simulink model "CAMFC2_Quad_New_02_Payload_01"  (R2018b)
settings: Solver=ode45  StartTime=0.0  StopTime=200  RelTol=1e-3  EnableMultiTasking=on
InitFcn:
  | constant_CAMFC2_Quad_New_02_Payload_01
values from neighbouring files (symbols this model uses):
  alpha = 0.01    [constant_CAMFC2_Quad_New_02_Payload_01.m]
  AN = [     0 1 0 0 ... (first row only)    [constant_CAMFC2_Quad_New_02_Payload_01.m]
  B = 1e0*eye(n)    [Simple_2Quad_payload_03_const.m]    (also in constant_CAMFC2_Quad_New_02_Payload_01.m = eye(n); test01.m = [eye(3) eye(3) eye(3) eye(3))
  B_pseudo_inverse = ((B'*B)^(-1))*B'    [constant_CAMFC2_Quad_New_02_Payload_01.m]
  BBT_inv = ((B'*B)^(-1))*B'    [Simple_2Quad_payload_03_const.m]    (also in Simple_4Quad_payload_04_const.m = ((BR'*BR)^(-1))*BR'; Simple_4Quad_payload_05_const.m = ((BR'*BR)^(-1))*BR'; Simple_4Quad_payload_06_const.m = ((BR'*BR)^(-1))*BR'; Simple_4Quad_payload_07_const.m = ((BR'*BR)^(-1))*BR')
  Beta = 0.1    [constant_CAMFC2_Quad_New_02_Payload_01.m]
  BN = [     1 0 0 0 ... (first row only)    [constant_CAMFC2_Quad_New_02_Payload_01.m]
  epsilon_struct = struct('data',epsilon_InitVal)    [constant_CAMFC2_Quad_New_02_Payload_01.m]
  gama1 = 1e+3*diag([1e-6*ones(n0,1);1e-0*ones(n0,1)])    [constant_CAMFC2_Quad_New_02_Payload_01.m]
  gama2 = 1e-1*diag([1e-6*ones(n0,1);1e-0*ones(n0,1)])    [constant_CAMFC2_Quad_New_02_Payload_01.m]
  gamma_0 = 1e-0*diag([1e-3;1e-0])    [Simple_2Quad_payload_03_const.m]    (also in Simple_4Quad_payload_04_const.m = 1e-0*diag([1e-6*ones(3,1);1e-0*ones(3,1)]); Simple_4Quad_payload_05_const.m = 1e-1*diag([1e-6*ones(3,1);1e-0*ones(3,1)]); Simple_4Quad_payload_06_const.m = 1e-0*diag([1e-6*ones(3,1);1e-0*ones(3,1)]); Simple_4Quad_payload_07_const.m = 1e-0*diag([1e-6*ones(3,1);1e-0*ones(3,1)]))
  gamma_1 = 1e+2*diag([1e-3;1e-0])    [Simple_2Quad_payload_03_const.m]    (also in Simple_4Quad_payload_04_const.m = 1e+2*diag([1e-6*ones(3,1);1e-0*ones(3,1)]); Simple_4Quad_payload_05_const.m = 1e+2*diag([1e-6*ones(3,1);1e-0*ones(3,1)]); Simple_4Quad_payload_06_const.m = 1e+3*diag([1e-6*ones(3,1);1e-0*ones(3,1)]); Simple_4Quad_payload_07_const.m = 1e+3*diag([1e-6*ones(3,1);1e-0*ones(3,1)]))
  ge = 9.81    [Simple_4Quad_payload_03_const.m]    (also in constant_CAMFC2_Quad_New_02_Payload_01.m)
  H = L + BN    [constant_CAMFC2_Quad_New_02_Payload_01.m]
  J = 1.2416e-3 * diag([1 1 2],0)    [constant_CAMFC2_Quad_New_02_Payload_01.m]
  K = 1e+1*eye(n)    [constant_CAMFC2_Quad_New_02_Payload_01.m]
  k1 = 1    [Simple_2Quad_payload_03_const.m]    (also in Simple_4Quad_payload_04_const.m; Simple_4Quad_payload_05_const.m; Simple_4Quad_payload_06_const.m; Simple_4Quad_payload_07_const.m)
  k2 = 0.1    [Simple_2Quad_payload_03_const.m]    (also in Simple_4Quad_payload_04_const.m; Simple_4Quad_payload_05_const.m; Simple_4Quad_payload_06_const.m; Simple_4Quad_payload_07_const.m)
  Ka = 0.01    [Simple_4Quad_payload_03_const.m]    (also in constant_CAMFC2_Quad_New_02_Payload_01.m)
  Kd = 0.01    [Simple_4Quad_payload_03_const.m]    (also in constant_CAMFC2_Quad_New_02_Payload_01.m)
  Kf = 1.0e-5    (= 1e-05)    [Simple_4Quad_payload_03_const.m]    (also in constant_CAMFC2_Quad_New_02_Payload_01.m)
  Kt = 0.0435 * Kf    (= 4.35e-07)    [Simple_4Quad_payload_03_const.m]    (also in constant_CAMFC2_Quad_New_02_Payload_01.m = 1e-07)
  Lq = 0.45    [Simple_4Quad_payload_03_const.m]    (also in constant_CAMFC2_Quad_New_02_Payload_01.m = 0.2)
  m = 1.5    [Colab_4Quad_model_01_const.m]    (also in Colab_4Quad_model_02_const.m; Simple_2Quad_payload_04_const.m = 1; Simple_4Quad_payload_01_const.m = 1; Simple_4Quad_payload_02_const.m = 1)
  M = 1.0    (= 1)    [Colab_4Quad_model_01_const.m]    (also in Colab_4Quad_model_02_const.m; Simple_2Quad_payload_01_const.m; Simple_2Quad_payload_02_const.m; Simple_2Quad_payload_03_const.m)
  mp = 10    [constant_CAMFC2_Quad_New_02_Payload_01.m]
  N = 4    [constant_CAMFC2_Quad_New_02_Payload_01.m]
  n = 2    [Simple_2Quad_payload_03_const.m]    (also in Simple_4Quad_payload_03_const.m = 6; Simple_4Quad_payload_04_const.m = 6; Simple_4Quad_payload_05_const.m = 6; Simple_4Quad_payload_06_const.m = 6)
  n0 = 3    [constant_CAMFC2_Quad_New_02_Payload_01.m]
  np = 3    [Simple_4Quad_payload_10_const.m]    (also in Simple_4Quad_payload_11_const.m; Simple_4Quad_payload_12_const.m; constant_CAMFC2_Quad_New_02_Payload_01.m = 6)
  Observer_Gain = 10    [constant_CAMFC2_Quad_New_02_Payload_01.m]
  Observer_Gain1 = 10    [constant_CAMFC2_Quad_New_02_Payload_01.m]
  P_struct = struct('data',P_InitVal)    [constant_CAMFC2_Quad_New_02_Payload_01.m]
  Q = 1e-1*eye(n)    [Simple_2Quad_payload_03_const.m]    (also in constant_CAMFC2_Quad_New_02_Payload_01.m = 1e+1*eye(n))
  QR = 1e-0*eye(n)    [Simple_4Quad_payload_04_const.m]    (also in Simple_4Quad_payload_05_const.m = 1e-1*eye(n); Simple_4Quad_payload_06_const.m; Simple_4Quad_payload_07_const.m; Simple_4Quad_payload_08_const.m)
  R = 1e+0*eye(n)    [Simple_2Quad_payload_03_const.m]    (also in Simple_4Quad_payload_04_const.m = 1e+0*eye(m); Simple_4Quad_payload_05_const.m = 1e+0*eye(m); Simple_4Quad_payload_06_const.m; Simple_4Quad_payload_07_const.m)
  r_formX = 1.0    (= 1)    [constant_CAMFC2_Quad_New_02_Payload_01.m]
  r_formY = 1.0    (= 1)    [constant_CAMFC2_Quad_New_02_Payload_01.m]
  r_formZ = 1.0    (= 1)    [constant_CAMFC2_Quad_New_02_Payload_01.m]
  rho1 = 1e-0    (= 1)    [constant_CAMFC2_Quad_New_02_Payload_01.m]
  rho2 = 1e-1    (= 0.1)    [constant_CAMFC2_Quad_New_02_Payload_01.m]
  rho_0 = 1e-0    (= 1)    [Simple_2Quad_payload_03_const.m]    (also in Simple_4Quad_payload_04_const.m; Simple_4Quad_payload_05_const.m = 0.1; Simple_4Quad_payload_06_const.m; Simple_4Quad_payload_07_const.m)
  rho_1 = 1e-0    (= 1)    [Simple_2Quad_payload_03_const.m]    (also in Simple_4Quad_payload_04_const.m; Simple_4Quad_payload_05_const.m; Simple_4Quad_payload_06_const.m; Simple_4Quad_payload_07_const.m)
  T_struct = struct('data',T_InitVal)    [constant_CAMFC2_Quad_New_02_Payload_01.m]
  U_dot0_M = U_dot0_m*ones(n0,1)    [constant_CAMFC2_Quad_New_02_Payload_01.m]
  Upsilon_M = Upsilon_m*ones(n0,1)    [constant_CAMFC2_Quad_New_02_Payload_01.m]
  X_M = X_m*ones(n0,1)    [constant_CAMFC2_Quad_New_02_Payload_01.m]
(part 1 of 3)
settings Model: ExtModeTrigDuration=100  Creator=hp  LastModifiedBy=ali
settings DataIOCC: LimitDataPoints=on  SaveFinalState=on  SaveFormat=StructureWithTime  SaveOutput=off  SaveState=on  StateSaveName=tmp_raccel_xout  SignalLoggingName=tmp_raccel_logsout
settings OptimizationCC: EfficientMapNaN2IntZero=off  LifeSpan=inf
settings DebuggingCC: UnderspecifiedInitializationDetection=Classic  MergeDetectMultiDrivingBlocksExec=none  SFUnexpectedBacktrackingDiag=warning  SFNoUnconditionalDefaultTransitionDiag=warning  SFExecutionAtInitializationDiag=none
settings HardwareCC: ProdBitPerPointer=32  ProdBitPerSizeT=32  ProdBitPerPtrDiffT=32  ProdLargestAtomicFloat=None  ProdIntDivRoundTo=Undefined  ProdEndianess=Unspecified  ProdWordSize=32  ProdHWDeviceType=32-bit Generic  TargetBitPerPointer=64  TargetBitPerSizeT=64  TargetBitPerPtrDiffT=64  TargetLongLongMode=on  TargetIntDivRoundTo=Zero  TargetEndianess=LittleEndian  TargetWordSize=64  TargetHWDeviceType=MATLAB Host  ProdEqTarget=off
settings ModelReferenceCC: PropagateSignalLabelsOutOfModel=off
settings SFSimCC: SimUseLocalCustomCode=off
settings RTWCC: SystemTargetFile=raccel.tlc  TemplateMakefile=raccel_default_tmf  RTWVerbose=off  RTWUseLocalCustomCode=off  RTWUseSimCustomCode=on
settings CodeAppCC: GenerateComments=off  MaxIdLength=128  MangleLength=10  SimulinkBlockComments=off
settings RaccelTargetCC: GeneratePreprocessorConditionals=Use local settings  MultiInstanceERTCode=off  PreserveStateflowLocalDataDimensions=off  ExtModeMexArgs='', 0, 54523  ENABLE_SLEXEC_SSBRIDGE=0  RTWCAPIParams=on
settings ConfigComp: CovMetricSettings=dw  CovHtmlReporting=on  CovSaveCumulativeToWorkspaceVar=on  CovSaveSingleToWorkspaceVar=on  CovExternalEMLEnable=off

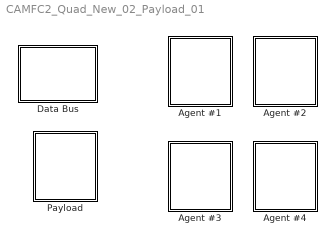
== system CAMFC2_Quad_New_02_Payload_01 ==
  Agent #1 : Subsystem
  Agent #2 : Subsystem
  Agent #3 : Subsystem
  Agent #4 : Subsystem
  "Data Bus " : Subsystem
  Payload : Subsystem

== system CAMFC2_Quad_New_02_Payload_01/Agent #1 ==
  Agent # : Constant
  Controller #1 : Subsystem
  Plant #1 : Subsystem
  tag scope: x1=global
  wires:
  Plant #1/1(X) -> [x1]
  Controller #1/1(u1) -> Plant #1/1(U)
  Agent #/1 -> Controller #1/1(Agent No.)

== system CAMFC2_Quad_New_02_Payload_01/Agent #2 ==
  Agent # : Constant  Value=2
  Controller #2 : Subsystem
  Plant #2 : Subsystem
  tag scope: x2=global
  wires:
  Plant #2/1(X) -> [x2]
  Controller #2/1(u2) -> Plant #2/1(U)
  Agent #/1 -> Controller #2/1(Agent No.)

== system CAMFC2_Quad_New_02_Payload_01/Agent #3 ==
  Agent # : Constant  Value=3
  Controller #3 : Subsystem
  Plant #3 : Subsystem
  tag scope: x3=global
  wires:
  Plant #3/1(X) -> [x3]
  Controller #3/1(u3) -> Plant #3/1(U)
  Agent #/1 -> Controller #3/1(Agent No.)

== system CAMFC2_Quad_New_02_Payload_01/Agent #4 ==
  Agent # : Constant  Value=4
  Controller #4 : Subsystem
  Plant #4 : Subsystem
  tag scope: x4=global
  wires:
  Plant #4/1(X) -> [x4]
  Controller #4/1(u4) -> Plant #4/1(U)
  Agent #/1 -> Controller #4/1(Agent No.)

== system CAMFC2_Quad_New_02_Payload_01/Data Bus  ==
  Mux6 : Mux
  Observers Log : Subsystem
  Reference Trajectory : Subsystem
  Rotational Log : Subsystem
  Scope{1..2,16..19,25..26} (8 alike) : Scope
  Sum : Sum  Inputs=|-+
  Translational Log : Subsystem
  formation of the leader : Constant  Value=zeros(n0,1)
  tag scope: u0=global, x0=global, x=global, z0=global
  wires:
  Reference Trajectory/2(U0) -> [u0], Scope25/1
  Reference Trajectory/1(X0) -> [x0], Sum/1, Scope26/1
  [x2] -> Scope17/1, Mux6/2
  [x1] -> Scope16/1, Mux6/1
  Mux6/1 -> [x]
  [x3] -> Scope18/1, Mux6/3
  [x4] -> Mux6/4, Scope19/1
  formation of the leader/1 -> Sum/2
  Sum/1 -> [z0]
  [x_p] -> Scope1/1
  [u_p] -> Scope2/1

== system CAMFC2_Quad_New_02_Payload_01/Payload ==
  "Controller " : Subsystem
  Plant : Subsystem
  tag scope: u_p=global, x_p=global
  wires:
  "Controller "/1(u) -> [u_p], Plant/1(U)
  Plant/1(X) -> "Controller "/1(X), [x_p]

== system CAMFC2_Quad_New_02_Payload_01/Agent #1/Controller #1 ==
  Agent No. : Inport
  Controller Interpreter #1 : MATLAB Function  TreatAsAtomicUnit=on
  Controller to Motors #1 : MATLAB Function  TreatAsAtomicUnit=on
  Cooperative Observers #1 : Subsystem
  Demux : Demux  Outputs=2
  Rotational : Subsystem
  Scope : Scope
  Sum : Sum  Inputs=|++
  Translational #1 : Subsystem
  u1 : Outport
  tag scope: u1=global
  wires:
  Controller Interpreter #1/2(PHI_d_i) -> Rotational/1(x_rd), Scope/1
  Controller Interpreter #1/1(uT_i) -> Controller to Motors #1/1(uT)
  Rotational/1(ur) -> Controller to Motors #1/2(uR)
  Controller to Motors #1/1(u) -> [u1], u1/1
  [x1] -> Rotational/2(X)
  Cooperative Observers #1/4(x0_hati) -> Translational #1/5(x0_hati)
  Translational #1/1(u1_T) -> Demux/1
  Cooperative Observers #1/1(Ti) -> Translational #1/2(Ti)
  Cooperative Observers #1/2(DTi) -> Translational #1/3(DTi)
  Cooperative Observers #1/3(qi) -> Translational #1/4(qi)
  Agent No./1 -> Translational #1/1(Agent No.), Cooperative Observers #1/1(Agent #)
  Sum/1 -> Controller Interpreter #1/1(ut_i)
  [upi] -> Sum/2
  Demux/2 -> Sum/1

== system CAMFC2_Quad_New_02_Payload_01/Agent #1/Plant #1 ==
  U : Inport
  Clock : Clock
  Integrator : Integrator  InitialCondition=zeros(2*n,1)
  MATLAB Function : MATLAB Function  TreatAsAtomicUnit=on
  X : Outport
  wires:
  Clock/1 -> MATLAB Function/3(t)
  MATLAB Function/1(DX) -> Integrator/1
  Integrator/1 -> MATLAB Function/1(X), X/1
  U/1 -> MATLAB Function/2(U)

== system CAMFC2_Quad_New_02_Payload_01/Agent #2/Controller #2 ==
  Agent No. : Inport
  Controller Interpreter #2 : MATLAB Function  TreatAsAtomicUnit=on
  Controller To Motors #2 : MATLAB Function  TreatAsAtomicUnit=on
  Cooperative Observers #2 : Subsystem
  Demux : Demux  Outputs=2
  Rotational : Subsystem
  Scope : Scope
  Sum : Sum  Inputs=|++
  Translational #2 : Subsystem
  u2 : Outport
  tag scope: u2=global
  wires:
  Controller Interpreter #2/2(PHI_d_i) -> Scope/1, Rotational/1(x_rd)
  Controller Interpreter #2/1(uT_i) -> Controller To Motors #2/1(uT)
  Rotational/1(ur) -> Controller To Motors #2/2(uR)
  Controller To Motors #2/1(u) -> [u2], u2/1
  [x2] -> Rotational/2(X)
  Cooperative Observers #2/3(qi) -> Translational #2/4(qi)
  Cooperative Observers #2/4(x0_hati) -> Translational #2/5(x0_hati)
  Translational #2/1(u2_T) -> Demux/1
  Agent No./1 -> Translational #2/1(Agent No.), Cooperative Observers #2/1(Agent #)
  Cooperative Observers #2/1(Ti) -> Translational #2/2(Ti)
  Cooperative Observers #2/2(DTi) -> Translational #2/3(DTi)
  Sum/1 -> Controller Interpreter #2/1(ut_i)
  [upi] -> Sum/2
  Demux/2 -> Sum/1

== system CAMFC2_Quad_New_02_Payload_01/Agent #2/Plant #2 ==
  U : Inport
  Clock : Clock
  Integrator : Integrator  InitialCondition=zeros(2*n,1)
  MATLAB Function : MATLAB Function  TreatAsAtomicUnit=on
  X : Outport
  wires:
  Clock/1 -> MATLAB Function/3(t)
  MATLAB Function/1(DX) -> Integrator/1
  Integrator/1 -> MATLAB Function/1(X), X/1
  U/1 -> MATLAB Function/2(U)

== system CAMFC2_Quad_New_02_Payload_01/Agent #3/Controller #3 ==
  Agent No. : Inport
  Controller Interpreter #3 : MATLAB Function  TreatAsAtomicUnit=on
  Controller to Motors #3 : MATLAB Function  TreatAsAtomicUnit=on
  Cooperative Observers #3 : Subsystem
  Demux : Demux  Outputs=2
  Rotational : Subsystem
  Scope : Scope
  Sum : Sum  Inputs=|++
  Translational #3 : Subsystem
  u3 : Outport
  tag scope: u3=global
  wires:
  Controller Interpreter #3/1(uT_i) -> Controller to Motors #3/1(uT)
  Rotational/1(ur) -> Controller to Motors #3/2(uR)
  Controller to Motors #3/1(u) -> [u3], u3/1
  Controller Interpreter #3/2(PHI_d_i) -> Scope/1, Rotational/1(x_rd)
  [x3] -> Rotational/2(X)
  Cooperative Observers #3/1(Ti) -> Translational #3/2(Ti)
  Cooperative Observers #3/2(DTi) -> Translational #3/3(DTi)
  Cooperative Observers #3/3(qi) -> Translational #3/4(qi)
  Cooperative Observers #3/4(x0_hati) -> Translational #3/5(x0_hati)
  Translational #3/1(u3_T) -> Demux/1
  Agent No./1 -> Translational #3/1(Agent No.), Cooperative Observers #3/1(Agent #)
  Sum/1 -> Controller Interpreter #3/1(ut_i)
  [upi] -> Sum/2
  Demux/2 -> Sum/1

== system CAMFC2_Quad_New_02_Payload_01/Agent #3/Plant #3 ==
  U : Inport
  Clock : Clock
  Integrator : Integrator  InitialCondition=zeros(2*n,1)
  MATLAB Function : MATLAB Function  TreatAsAtomicUnit=on
  X : Outport
  wires:
  Clock/1 -> MATLAB Function/3(t)
  MATLAB Function/1(DX) -> Integrator/1
  Integrator/1 -> MATLAB Function/1(X), X/1
  U/1 -> MATLAB Function/2(U)

== system CAMFC2_Quad_New_02_Payload_01/Agent #4/Controller #4 ==
  Agent No. : Inport
  Controller Interpreter #4 : MATLAB Function  TreatAsAtomicUnit=on
  Controller to Motors #4 : MATLAB Function  TreatAsAtomicUnit=on
  Cooperative Observers #1 : Subsystem
  Demux : Demux  Outputs=2
  Rotational : Subsystem
  Scope : Scope
  Sum : Sum  Inputs=|++
  Translational #4 : Subsystem
  u4 : Outport
  tag scope: u4=global
  wires:
  Controller Interpreter #4/2(PHI_d_i) -> Rotational/1(x_rd), Scope/1
  Controller Interpreter #4/1(uT_i) -> Controller to Motors #4/1(uT)
  Rotational/1(ur) -> Controller to Motors #4/2(uR)
  Controller to Motors #4/1(u) -> [u4], u4/1
  [x4] -> Rotational/2(X)
  Cooperative Observers #1/2(DTi) -> Translational #4/3(DTi)
  Agent No./1 -> Translational #4/1(Agent No.), Cooperative Observers #1/1(Agent #)
  Cooperative Observers #1/3(qi) -> Translational #4/4(qi)
  Translational #4/1(u4_T) -> Demux/1
  Cooperative Observers #1/4(x0_hati) -> Translational #4/5(x0_hati)
  Cooperative Observers #1/1(Ti) -> Translational #4/2(Ti)
  Sum/1 -> Controller Interpreter #4/1(ut_i)
  Demux/2 -> Sum/1
  [upi] -> Sum/2

== system CAMFC2_Quad_New_02_Payload_01/Agent #4/Plant #4 ==
  U : Inport
  Clock : Clock
  Integrator : Integrator  InitialCondition=zeros(2*n,1)
  MATLAB Function : MATLAB Function  TreatAsAtomicUnit=on
  X : Outport
  wires:
  Clock/1 -> MATLAB Function/3(t)
  MATLAB Function/1(DX) -> Integrator/1
  Integrator/1 -> MATLAB Function/1(X), X/1
  U/1 -> MATLAB Function/2(U)

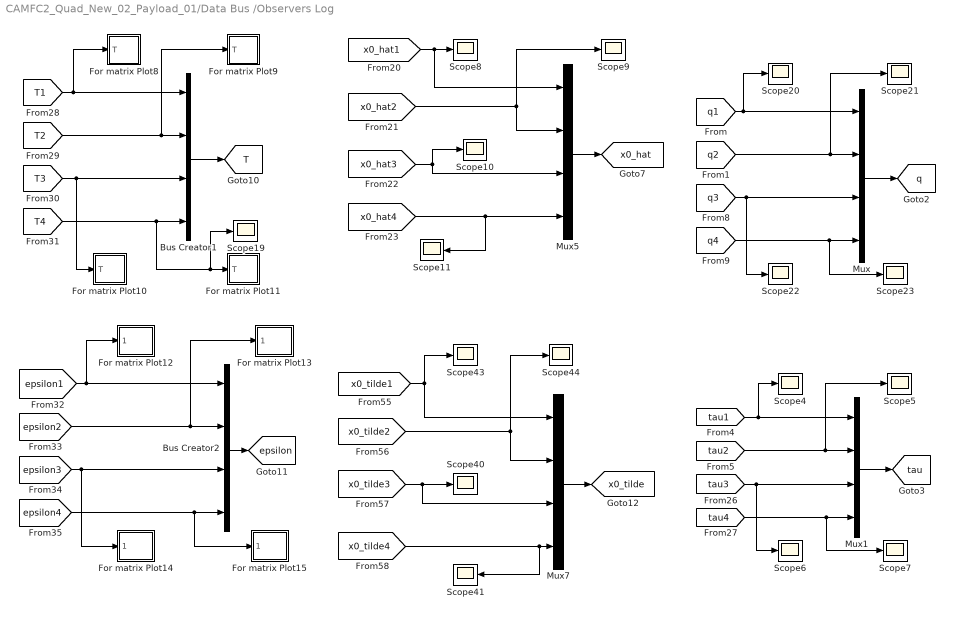
== system CAMFC2_Quad_New_02_Payload_01/Data Bus /Observers Log ==
  Bus Creator1 : BusCreator  Inputs=4  OutDataTypeStr=Bus: T_bus
  Bus Creator2 : BusCreator  Inputs=4  OutDataTypeStr=Bus: epsilon_bus
  For matrix Plot10 : Subsystem
  For matrix Plot11 : Subsystem
  For matrix Plot12 : Subsystem
  For matrix Plot13 : Subsystem
  For matrix Plot14 : Subsystem
  For matrix Plot15 : Subsystem
  For matrix Plot8 : Subsystem
  For matrix Plot9 : Subsystem
  Mux{,1,5,7} (4 alike) : Mux
  Scope{4..11,19..23,40..41,43..44} (17 alike) : Scope
  tag scope: T=global, epsilon=global, q=global, tau=global, x0_hat=global, x0_tilde=global
  wires:
  [epsilon4] -> For matrix Plot15/1(epsilon), Bus Creator2/4
  [x0_tilde1] -> Scope43/1, Mux7/1
  [epsilon1] -> For matrix Plot12/1(epsilon), Bus Creator2/1
  [T2] -> For matrix Plot9/1(T), Bus Creator1/2
  Mux7/1 -> [x0_tilde]
  [x0_tilde3] -> Mux7/3, Scope40/1
  Bus Creator2/1 -> [epsilon]
  [T3] -> For matrix Plot10/1(T), Bus Creator1/3
  [x0_tilde2] -> Scope44/1, Mux7/2
  [epsilon3] -> For matrix Plot14/1(epsilon), Bus Creator2/3
  [T4] -> Scope19/1, For matrix Plot11/1(T), Bus Creator1/4
  [x0_tilde4] -> Scope41/1, Mux7/4
  [epsilon2] -> For matrix Plot13/1(epsilon), Bus Creator2/2
  [T1] -> For matrix Plot8/1(T), Bus Creator1/1
  Bus Creator1/1 -> [T]
  [x0_hat1] -> Scope8/1, Mux5/1
  [q4] -> Scope23/1, Mux/4
  [x0_hat4] -> Mux5/4, Scope11/1
  [x0_hat3] -> Scope10/1, Mux5/3
  [x0_hat2] -> Scope9/1, Mux5/2
  Mux/1 -> [q]
  Mux5/1 -> [x0_hat]
  [q1] -> Scope20/1, Mux/1
  [q2] -> Scope21/1, Mux/2
  [q3] -> Scope22/1, Mux/3
  [tau4] -> Scope7/1, Mux1/4
  [tau3] -> Scope6/1, Mux1/3
  Mux1/1 -> [tau]
  [tau2] -> Scope5/1, Mux1/2
  [tau1] -> Scope4/1, Mux1/1

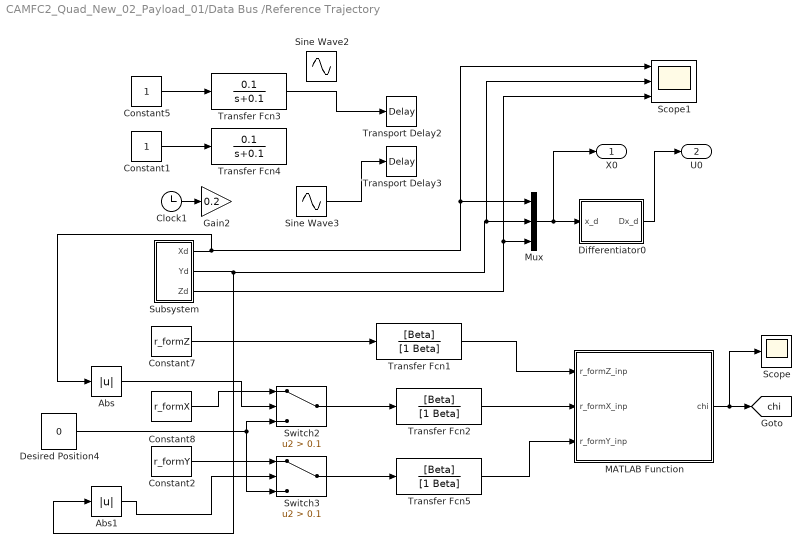
== system CAMFC2_Quad_New_02_Payload_01/Data Bus /Reference Trajectory ==
  Abs : Abs
  Abs1 : Abs
  Clock1 : Clock
  Constant1 : Constant
  Constant2 : Constant  Value=r_formY
  Constant5 : Constant
  Constant7 : Constant  Value=r_formZ
  Constant8 : Constant  Value=r_formX
  Desired Position4 : Constant  Value=0  VectorParams1D=off
  Differentiator0 : Subsystem
  Gain2 : Gain  Gain=0.2
  MATLAB Function : MATLAB Function  TreatAsAtomicUnit=on
  Mux : Mux  Inputs=3
  Scope : Scope
  Scope1 : Scope  NumInputPorts=3
  Sine Wave2 : Sin  Amplitude=3  Bias=-3  Frequency=0.1  Phase=pi/2  SampleTime=0
  Sine Wave3 : Sin  Amplitude=3  Frequency=0.1  SampleTime=0
  Subsystem : Subsystem
  Switch2 : Switch  Criteria=u2 > Threshold  Threshold=0.1
  Switch3 : Switch  Criteria=u2 > Threshold  Threshold=0.1
  Transfer Fcn1 : TransferFcn  Numerator=[Beta]  Denominator=[1 Beta]
  Transfer Fcn2 : TransferFcn  Numerator=[Beta]  Denominator=[1 Beta]
  Transfer Fcn3 : TransferFcn  Numerator=[0.1]  Denominator=[1 0.1]
  Transfer Fcn4 : TransferFcn  Numerator=[0.1]  Denominator=[1 0.1]
  Transfer Fcn5 : TransferFcn  Numerator=[Beta]  Denominator=[1 Beta]
  Transport Delay2 : TransportDelay  DelayTime=20
  Transport Delay3 : TransportDelay  DelayTime=20
  X0 : Outport
  U0 : Outport  Port=2
  tag scope: chi=global
  wires:
  Subsystem/1(Xd) -> Scope1/1, Mux/1, Abs/1
  Differentiator0/1(Dx_d) -> U0/1
  Mux/1 -> Differentiator0/1(x_d), X0/1
  MATLAB Function/1(chi) -> Scope/1, [chi]
  Transfer Fcn1/1 -> MATLAB Function/1(r_formZ_inp)
  Transfer Fcn2/1 -> MATLAB Function/2(r_formX_inp)
  Constant5/1 -> Transfer Fcn3/1
  Clock1/1 -> Gain2/1
  Subsystem/2(Yd) -> Scope1/2, Mux/2, Abs1/1
  Constant1/1 -> Transfer Fcn4/1
  Sine Wave3/1 -> Transport Delay3/1
  Switch3/1 -> Transfer Fcn5/1
  Transfer Fcn5/1 -> MATLAB Function/3(r_formY_inp)
  Transfer Fcn3/1 -> Transport Delay2/1
  Switch2/1 -> Transfer Fcn2/1
  Constant7/1 -> Transfer Fcn1/1
  Subsystem/3(Zd) -> Scope1/3, Mux/3
  Abs/1 -> Switch2/2
  Constant8/1 -> Switch2/1
  Desired Position4/1 -> Switch2/3, Switch3/3
  Constant2/1 -> Switch3/1
  Abs1/1 -> Switch3/2

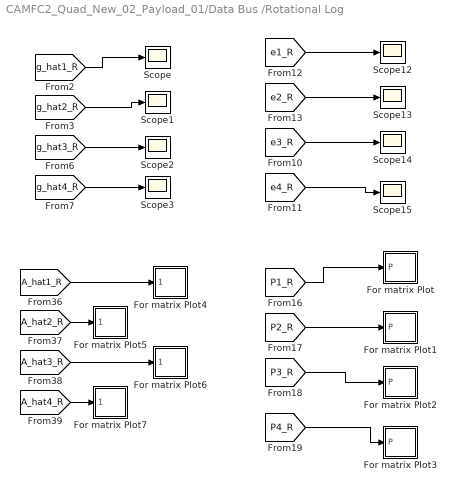
== system CAMFC2_Quad_New_02_Payload_01/Data Bus /Rotational Log ==
  For matrix Plot : Subsystem
  For matrix Plot1 : Subsystem
  For matrix Plot2 : Subsystem
  For matrix Plot3 : Subsystem
  For matrix Plot4 : Subsystem
  For matrix Plot5 : Subsystem
  For matrix Plot6 : Subsystem
  For matrix Plot7 : Subsystem
  Scope{,1..3,12..15} (8 alike) : Scope
  wires:
  [g_hat1_R] -> Scope/1
  [g_hat3_R] -> Scope2/1
  [g_hat2_R] -> Scope1/1
  [g_hat4_R] -> Scope3/1
  [e2_R] -> Scope13/1
  [P1_R] -> For matrix Plot/1(P)
  [e4_R] -> Scope15/1
  [P4_R] -> For matrix Plot3/1(P)
  [e3_R] -> Scope14/1
  [P3_R] -> For matrix Plot2/1(P)
  [e1_R] -> Scope12/1
  [P2_R] -> For matrix Plot1/1(P)
  [A_hat4_R] -> For matrix Plot7/1(A_hat)
  [A_hat2_R] -> For matrix Plot5/1(A_hat)
  [A_hat1_R] -> For matrix Plot4/1(A_hat)
  [A_hat3_R] -> For matrix Plot6/1(A_hat)

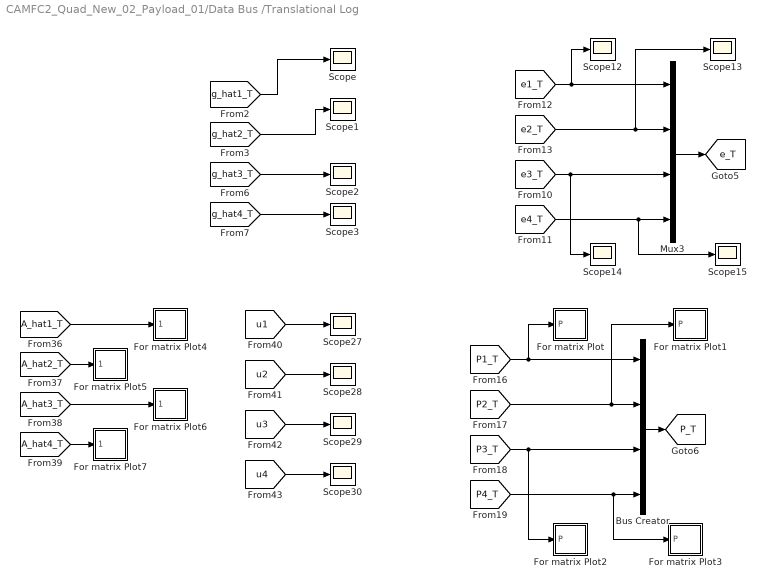
== system CAMFC2_Quad_New_02_Payload_01/Data Bus /Translational Log ==
  Bus Creator : BusCreator  Inputs=4  OutDataTypeStr=Bus: P_bus
  For matrix Plot : Subsystem
  For matrix Plot1 : Subsystem
  For matrix Plot2 : Subsystem
  For matrix Plot3 : Subsystem
  For matrix Plot4 : Subsystem
  For matrix Plot5 : Subsystem
  For matrix Plot6 : Subsystem
  For matrix Plot7 : Subsystem
  Mux3 : Mux
  Scope{,1..3,12..15,27..30} (12 alike) : Scope
  tag scope: P_T=global, e_T=global
  wires:
  [A_hat3_T] -> For matrix Plot6/1(A_hat)
  [A_hat1_T] -> For matrix Plot4/1(A_hat)
  [A_hat2_T] -> For matrix Plot5/1(A_hat)
  [A_hat4_T] -> For matrix Plot7/1(A_hat)
  [P2_T] -> For matrix Plot1/1(P), Bus Creator/2
  [e1_T] -> Scope12/1, Mux3/1
  [P3_T] -> For matrix Plot2/1(P), Bus Creator/3
  [e3_T] -> Scope14/1, Mux3/3
  Bus Creator/1 -> [P_T]
  [P4_T] -> For matrix Plot3/1(P), Bus Creator/4
  [e4_T] -> Mux3/4, Scope15/1
  [P1_T] -> For matrix Plot/1(P), Bus Creator/1
  [e2_T] -> Scope13/1, Mux3/2
  Mux3/1 -> [e_T]
  [u2] -> Scope28/1
  [u3] -> Scope29/1
  [u1] -> Scope27/1
  [u4] -> Scope30/1
  [g_hat4_T] -> Scope3/1
  [g_hat2_T] -> Scope1/1
  [g_hat3_T] -> Scope2/1
  [g_hat1_T] -> Scope/1

== system CAMFC2_Quad_New_02_Payload_01/Payload/Controller  ==
  X : Inport
  Constant : Constant  Value=0
  Constant1 : Constant  Value=0
  Constant2 : Constant  Value=2
  Control law : MATLAB Function  TreatAsAtomicUnit=on
  Demux : Demux  Outputs=2
  Derivative : Derivative
  Derivative1 : Derivative
  Gain : Gain  Gain=1/4
  Integrator : Integrator
  Mux : Mux  Inputs=3
  Scope : Scope
  Sum : Sum  Inputs=|+-
  u : Outport
  tag scope: upi=global
  wires:
  Control law/1(u) -> u/1, Gain/1
  X/1 -> Demux/1
  Demux/2 -> Control law/5(v)
  Constant2/1 -> Mux/3
  Constant1/1 -> Mux/2
  Constant/1 -> Mux/1
  [x0] -> Derivative/1, Sum/1
  Demux/1 -> Sum/2
  Sum/1 -> Control law/3(e), Scope/1, Integrator/1
  Gain/1 -> [upi]
  Derivative/1 -> Control law/2(Dp_d), Derivative1/1
  Derivative1/1 -> Control law/1(DDp_d)
  Integrator/1 -> Control law/4(Ie)

== system CAMFC2_Quad_New_02_Payload_01/Payload/Plant ==
  U : Inport
  Integrator : Integrator  InitialCondition=zeros(np,1)
  MATLAB Function : MATLAB Function  TreatAsAtomicUnit=on
  X : Outport
  wires:
  U/1 -> MATLAB Function/2(U)
  Integrator/1 -> X/1, MATLAB Function/1(X)
  MATLAB Function/1(DX) -> Integrator/1

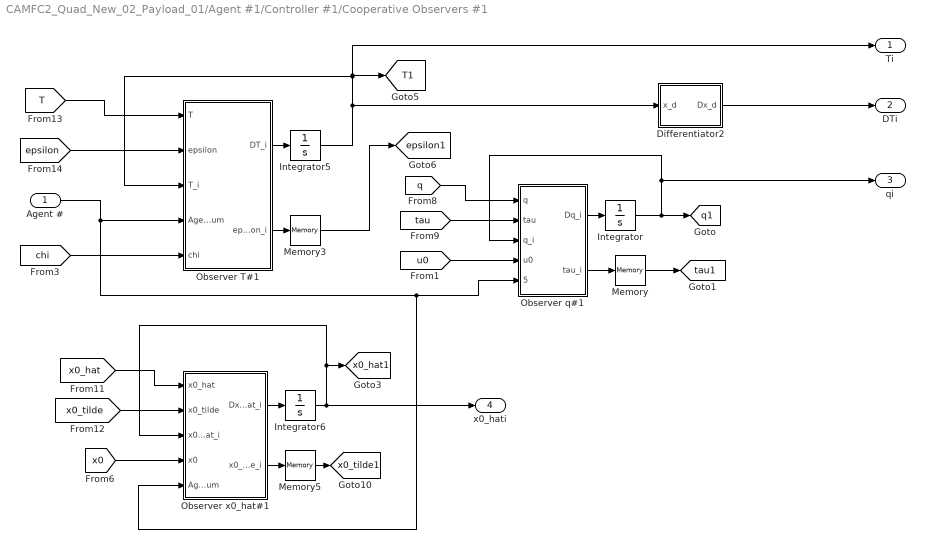
== system CAMFC2_Quad_New_02_Payload_01/Agent #1/Controller #1/Cooperative Observers #1 ==
  Agent # : Inport
  Differentiator2 : Subsystem
  Integrator : Integrator  InitialCondition=zeros(n0,1)
  Integrator5 : Integrator  InitialCondition=zeros(N+1,n0)
  Integrator6 : Integrator  InitialCondition=zeros(n0,1)
  Memory : Memory  InitialCondition=zeros(n0,1)
  Memory3 : Memory  InitialCondition=zeros(N+1,n0)
  Memory5 : Memory  InitialCondition=zeros(n0,1)
  Observer T#1 : MATLAB Function  TreatAsAtomicUnit=on
  Observer q#1 : MATLAB Function  TreatAsAtomicUnit=on
  Observer x0_hat#1 : MATLAB Function  TreatAsAtomicUnit=on
  Ti : Outport
  DTi : Outport  Port=2
  qi : Outport  Port=3
  x0_hati : Outport  Port=4
  tag scope: T1=global, epsilon1=global, q1=global, tau1=global, x0_hat1=global, x0_tilde1=global
  wires:
  [x0_tilde] -> Observer x0_hat#1/2(x0_tilde)
  Agent #/1 -> Observer x0_hat#1/5(Agent_Num), Observer q#1/5(Agent_Num), Observer T#1/4(Agent_Num)
  Observer T#1/1(DT_i) -> Integrator5/1
  Integrator/1 -> [q1], qi/1, Observer q#1/3(q_i)
  [q] -> Observer q#1/1(q)
  Observer q#1/1(Dq_i) -> Integrator/1
  Observer T#1/2(epsilon_i) -> Memory3/1
  [x0] -> Observer x0_hat#1/4(x0)
  [x0_hat] -> Observer x0_hat#1/1(x0_hat)
  [chi] -> Observer T#1/5(chi)
  Integrator5/1 -> Ti/1, [T1], Observer T#1/3(T_i), Differentiator2/1(x_d)
  [T] -> Observer T#1/1(T)
  Observer x0_hat#1/1(Dx0_hat_i) -> Integrator6/1
  [epsilon] -> Observer T#1/2(epsilon)
  [tau] -> Observer q#1/2(tau)
  Memory5/1 -> [x0_tilde1]
  Observer x0_hat#1/2(x0_tilde_i) -> Memory5/1
  Integrator6/1 -> x0_hati/1, Observer x0_hat#1/3(x0_hat_i), [x0_hat1]
  Memory3/1 -> [epsilon1]
  Memory/1 -> [tau1]
  Observer q#1/2(tau_i) -> Memory/1
  [u0] -> Observer q#1/4(u0)
  Differentiator2/1(Dx_d) -> DTi/1

== system CAMFC2_Quad_New_02_Payload_01/Agent #1/Controller #1/Rotational ==
  x_rd : Inport
  X : Inport  Port=2
  CARE : MATLAB Function  TreatAsAtomicUnit=on
  Differentiator : Subsystem
  Integrator : Integrator  InitialCondition=zeros(n)
  Integrator1 : Integrator  InitialCondition=eye(n)
  Integrator2 : Integrator  InitialCondition=zeros(n,1)
  Integrator3 : Integrator  InitialCondition=zeros(n,1)
  Memory : Memory  InitialCondition=zeros(m,1)
  Scope10 : Scope
  Sum : Sum  Inputs=|++
  g-Estimator : MATLAB Function  TreatAsAtomicUnit=on
  g-Estimator1 : MATLAB Function  TreatAsAtomicUnit=on
  main : MATLAB Function  TreatAsAtomicUnit=on
  variable change : MATLAB Function  TreatAsAtomicUnit=on
  ur : Outport
  tag scope: A_hat1_R=global, P1_R=global, e1_R=global, g_hat1_R=global
  wires:
  x_rd/1 -> variable change/2(Xd)
  X/1 -> variable change/1(X)
  CARE/1(DP) -> Integrator1/1
  Sum/1 -> main/1(sigma), Scope10/1, g-Estimator/1(sigma), g-Estimator1/1(sigma)
  g-Estimator1/1(Da_hat) -> Integrator/1
  variable change/1(x_mod) -> main/7(x), g-Estimator1/2(x)
  Integrator1/1 -> g-Estimator1/3(P), CARE/1(P), [P1_R], g-Estimator/3(P), main/4(P)
  Integrator/1 -> [A_hat1_R], g-Estimator1/4(a_hat), CARE/2(a_hat), main/5(a_hat)
  g-Estimator/1(Dg_hat) -> Integrator2/1
  Differentiator/1(Dx_d) -> main/3(Dy_d)
  main/1(u) -> Memory/1, ur/1
  Integrator3/1 -> main/2(zeta), Sum/1
  variable change/2(xd_mod) -> Differentiator/1(x_d)
  variable change/3(e_mod) -> [e1_R], Sum/2, Integrator3/1
  Memory/1 -> variable change/3(u)
  Integrator2/1 -> main/6(g_hat), [g_hat1_R], g-Estimator/2(g_hat)

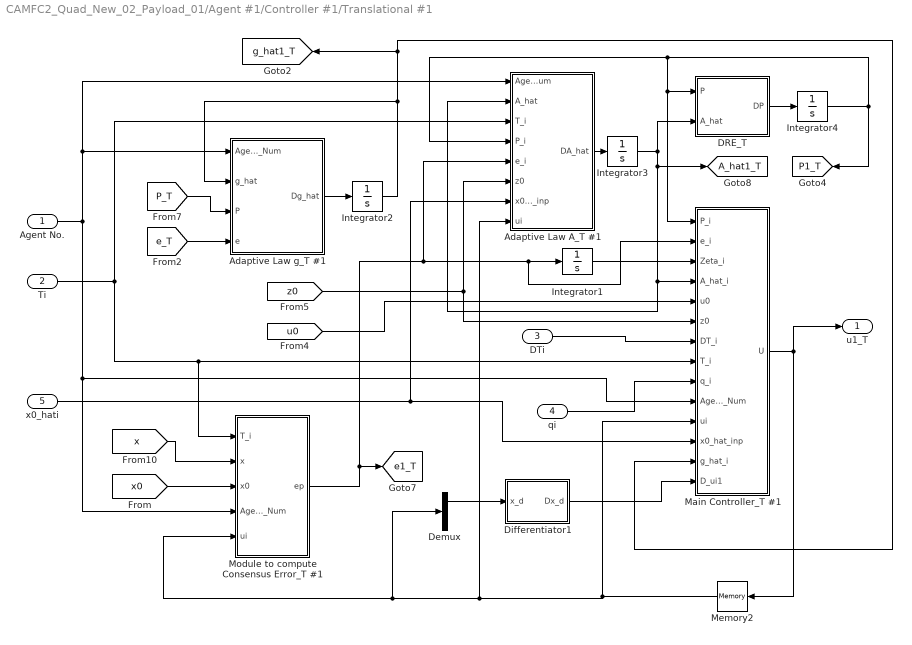
== system CAMFC2_Quad_New_02_Payload_01/Agent #1/Controller #1/Translational #1 ==
  Agent No. : Inport
  Ti : Inport  Port=2
  DTi : Inport  Port=3
  qi : Inport  Port=4
  x0_hati : Inport  Port=5
  Adaptive Law A_T #1 : MATLAB Function  TreatAsAtomicUnit=on
  Adaptive Law g_T #1 : MATLAB Function  TreatAsAtomicUnit=on
  DRE_T : MATLAB Function  TreatAsAtomicUnit=on
  Demux : Demux  Outputs=2
  Differentiator1 : Subsystem
  Integrator1 : Integrator  InitialCondition=zeros(n,1)
  Integrator2 : Integrator  InitialCondition=zeros(n,1)
  Integrator3 : Integrator  InitialCondition=zeros(n)
  Integrator4 : Integrator  InitialCondition=eye(n)
  Main Controller_T #1 : MATLAB Function  TreatAsAtomicUnit=on
  Memory2 : Memory  InitialCondition=zeros(n,1)
  Module to compute Consensus Error_T #1 : MATLAB Function  TreatAsAtomicUnit=on
  u1_T : Outport
  tag scope: A_hat1_T=global, P1_T=global, e1_T=global, g_hat1_T=global
  wires:
  [u0] -> Main Controller_T #1/5(u0)
  DRE_T/1(DP) -> Integrator4/1
  Module to compute Consensus Error_T #1/1(ep) -> Adaptive Law A_T #1/5(e_i), Main Controller_T #1/2(e_i), Integrator1/1, [e1_T]
  Adaptive Law g_T #1/1(Dg_hat) -> Integrator2/1
  Demux/1 -> Differentiator1/1(x_d)
  Main Controller_T #1/1(U) -> u1_T/1, Memory2/1
  Memory2/1 -> Adaptive Law A_T #1/8(ui), Module to compute Consensus Error_T #1/5(ui), Demux/1, Main Controller_T #1/11(ui)
  Adaptive Law A_T #1/1(DA_hat) -> Integrator3/1
  Integrator2/1 -> Main Controller_T #1/13(g_hat_i), [g_hat1_T], Adaptive Law g_T #1/2(g_hat)
  [e_T] -> Adaptive Law g_T #1/4(e)
  Integrator1/1 -> Main Controller_T #1/3(Zeta_i)
  Integrator3/1 -> [A_hat1_T], Adaptive Law A_T #1/2(A_hat), Main Controller_T #1/4(A_hat_i), DRE_T/2(A_hat)
  Integrator4/1 -> [P1_T], Adaptive Law A_T #1/4(P_i), DRE_T/1(P), Main Controller_T #1/1(P_i)
  [P_T] -> Adaptive Law g_T #1/3(P)
  [x0] -> Module to compute Consensus Error_T #1/3(x0)
  [x] -> Module to compute Consensus Error_T #1/2(x)
  [z0] -> Adaptive Law A_T #1/6(z0), Main Controller_T #1/6(z0)
  Agent No./1 -> Main Controller_T #1/10(Agent_Num), Module to compute Consensus Error_T #1/4(Agent_Num), Adaptive Law A_T #1/1(Agent_Num), Adaptive Law g_T #1/1(Agent_Num)
  Ti/1 -> Adaptive Law A_T #1/3(T_i), Module to compute Consensus Error_T #1/1(T_i), Main Controller_T #1/8(T_i)
  x0_hati/1 -> Adaptive Law A_T #1/7(x0_hat_inp), Main Controller_T #1/12(x0_hat_inp)
  DTi/1 -> Main Controller_T #1/7(DT_i)
  qi/1 -> Main Controller_T #1/9(q_i)
  Differentiator1/1(Dx_d) -> Main Controller_T #1/14(D_ui1)

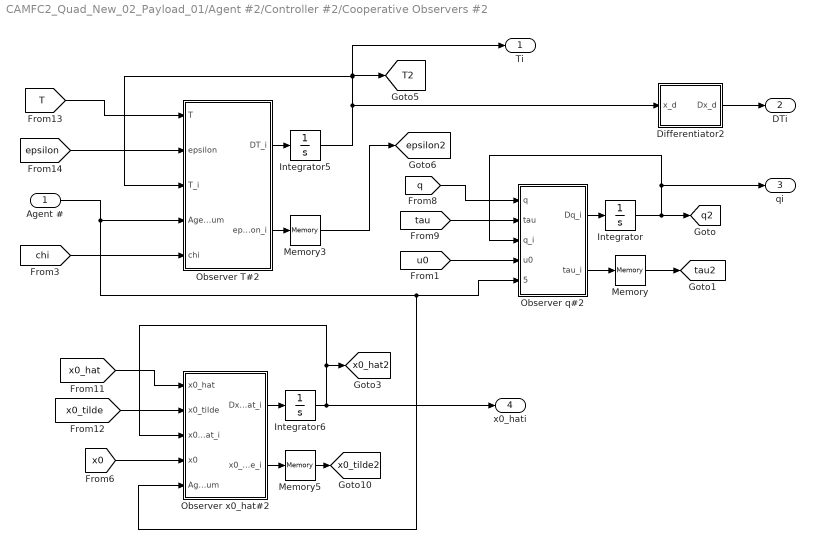
== system CAMFC2_Quad_New_02_Payload_01/Agent #2/Controller #2/Cooperative Observers #2 ==
  Agent # : Inport
  Differentiator2 : Subsystem
  Integrator : Integrator  InitialCondition=zeros(n0,1)
  Integrator5 : Integrator  InitialCondition=zeros(N+1,n0)
  Integrator6 : Integrator  InitialCondition=zeros(n0,1)
  Memory : Memory  InitialCondition=zeros(n0,1)
  Memory3 : Memory  InitialCondition=zeros(N+1,n0)
  Memory5 : Memory  InitialCondition=zeros(n0,1)
  Observer T#2 : MATLAB Function  TreatAsAtomicUnit=on
  Observer q#2 : MATLAB Function  TreatAsAtomicUnit=on
  Observer x0_hat#2 : MATLAB Function  TreatAsAtomicUnit=on
  Ti : Outport
  DTi : Outport  Port=2
  qi : Outport  Port=3
  x0_hati : Outport  Port=4
  tag scope: T2=global, epsilon2=global, q2=global, tau2=global, x0_hat2=global, x0_tilde2=global
  wires:
  [x0_tilde] -> Observer x0_hat#2/2(x0_tilde)
  Agent #/1 -> Observer q#2/5(Agent_Num), Observer x0_hat#2/5(Agent_Num), Observer T#2/4(Agent_Num)
  Observer T#2/1(DT_i) -> Integrator5/1
  Integrator/1 -> [q2], qi/1, Observer q#2/3(q_i)
  [q] -> Observer q#2/1(q)
  Observer q#2/1(Dq_i) -> Integrator/1
  Observer T#2/2(epsilon_i) -> Memory3/1
  [x0] -> Observer x0_hat#2/4(x0)
  [x0_hat] -> Observer x0_hat#2/1(x0_hat)
  [chi] -> Observer T#2/5(chi)
  Integrator5/1 -> Ti/1, [T2], Observer T#2/3(T_i), Differentiator2/1(x_d)
  [T] -> Observer T#2/1(T)
  Observer x0_hat#2/1(Dx0_hat_i) -> Integrator6/1
  [epsilon] -> Observer T#2/2(epsilon)
  [tau] -> Observer q#2/2(tau)
  Memory5/1 -> [x0_tilde2]
  Observer x0_hat#2/2(x0_tilde_i) -> Memory5/1
  Integrator6/1 -> x0_hati/1, Observer x0_hat#2/3(x0_hat_i), [x0_hat2]
  Memory3/1 -> [epsilon2]
  Memory/1 -> [tau2]
  Observer q#2/2(tau_i) -> Memory/1
  [u0] -> Observer q#2/4(u0)
  Differentiator2/1(Dx_d) -> DTi/1

== system CAMFC2_Quad_New_02_Payload_01/Agent #2/Controller #2/Rotational ==
  x_rd : Inport
  X : Inport  Port=2
  CARE : MATLAB Function  TreatAsAtomicUnit=on
  Differentiator : Subsystem
  Integrator : Integrator  InitialCondition=zeros(n)
  Integrator1 : Integrator  InitialCondition=eye(n)
  Integrator2 : Integrator  InitialCondition=zeros(n,1)
  Integrator3 : Integrator  InitialCondition=zeros(n,1)
  Memory : Memory  InitialCondition=zeros(m,1)
  Scope10 : Scope
  Sum : Sum  Inputs=|++
  g-Estimator : MATLAB Function  TreatAsAtomicUnit=on
  g-Estimator1 : MATLAB Function  TreatAsAtomicUnit=on
  main : MATLAB Function  TreatAsAtomicUnit=on
  variable change : MATLAB Function  TreatAsAtomicUnit=on
  ur : Outport
  tag scope: A_hat2_R=global, P2_R=global, e2_R=global, g_hat2_R=global
  wires:
  x_rd/1 -> variable change/2(Xd)
  X/1 -> variable change/1(X)
  CARE/1(DP) -> Integrator1/1
  Sum/1 -> main/1(sigma), Scope10/1, g-Estimator/1(sigma), g-Estimator1/1(sigma)
  g-Estimator1/1(Da_hat) -> Integrator/1
  variable change/1(x_mod) -> main/7(x), g-Estimator1/2(x)
  Integrator1/1 -> g-Estimator1/3(P), CARE/1(P), [P2_R], g-Estimator/3(P), main/4(P)
  Integrator/1 -> [A_hat2_R], g-Estimator1/4(a_hat), CARE/2(a_hat), main/5(a_hat)
  g-Estimator/1(Dg_hat) -> Integrator2/1
  Differentiator/1(Dx_d) -> main/3(Dy_d)
  main/1(u) -> Memory/1, ur/1
  Integrator3/1 -> main/2(zeta), Sum/1
  variable change/2(xd_mod) -> Differentiator/1(x_d)
  variable change/3(e_mod) -> [e2_R], Sum/2, Integrator3/1
  Memory/1 -> variable change/3(u)
  Integrator2/1 -> main/6(g_hat), [g_hat2_R], g-Estimator/2(g_hat)

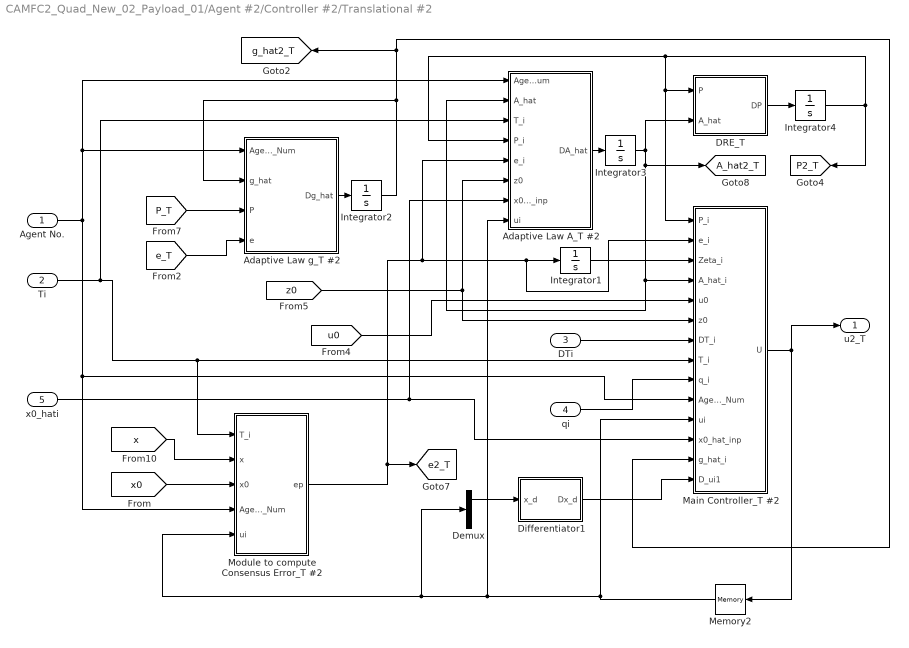
== system CAMFC2_Quad_New_02_Payload_01/Agent #2/Controller #2/Translational #2 ==
  Agent No. : Inport
  Ti : Inport  Port=2
  DTi : Inport  Port=3
  qi : Inport  Port=4
  x0_hati : Inport  Port=5
  Adaptive Law A_T #2 : MATLAB Function  TreatAsAtomicUnit=on
  Adaptive Law g_T #2 : MATLAB Function  TreatAsAtomicUnit=on
  DRE_T : MATLAB Function  TreatAsAtomicUnit=on
  Demux : Demux  Outputs=2
  Differentiator1 : Subsystem
  Integrator1 : Integrator  InitialCondition=zeros(n,1)
  Integrator2 : Integrator  InitialCondition=zeros(n,1)
  Integrator3 : Integrator  InitialCondition=zeros(n)
  Integrator4 : Integrator  InitialCondition=eye(n)
  Main Controller_T #2 : MATLAB Function  TreatAsAtomicUnit=on
  Memory2 : Memory  InitialCondition=zeros(n,1)
  Module to compute Consensus Error_T #2 : MATLAB Function  TreatAsAtomicUnit=on
  u2_T : Outport
  tag scope: A_hat2_T=global, P2_T=global, e2_T=global, g_hat2_T=global
  wires:
  [u0] -> Main Controller_T #2/5(u0)
  DRE_T/1(DP) -> Integrator4/1
  Module to compute Consensus Error_T #2/1(ep) -> Adaptive Law A_T #2/5(e_i), Main Controller_T #2/2(e_i), Integrator1/1, [e2_T]
  Adaptive Law g_T #2/1(Dg_hat) -> Integrator2/1
  Demux/1 -> Differentiator1/1(x_d)
  Main Controller_T #2/1(U) -> u2_T/1, Memory2/1
  Memory2/1 -> Main Controller_T #2/11(ui), Adaptive Law A_T #2/8(ui), Module to compute Consensus Error_T #2/5(ui), Demux/1
  Adaptive Law A_T #2/1(DA_hat) -> Integrator3/1
  Integrator2/1 -> Main Controller_T #2/13(g_hat_i), [g_hat2_T], Adaptive Law g_T #2/2(g_hat)
  [e_T] -> Adaptive Law g_T #2/4(e)
  Integrator1/1 -> Main Controller_T #2/3(Zeta_i)
  Integrator3/1 -> [A_hat2_T], Adaptive Law A_T #2/2(A_hat), Main Controller_T #2/4(A_hat_i), DRE_T/2(A_hat)
  Integrator4/1 -> [P2_T], Adaptive Law A_T #2/4(P_i), DRE_T/1(P), Main Controller_T #2/1(P_i)
  [P_T] -> Adaptive Law g_T #2/3(P)
  [x0] -> Module to compute Consensus Error_T #2/3(x0)
  [x] -> Module to compute Consensus Error_T #2/2(x)
  [z0] -> Adaptive Law A_T #2/6(z0), Main Controller_T #2/6(z0)
  Agent No./1 -> Main Controller_T #2/10(Agent_Num), Module to compute Consensus Error_T #2/4(Agent_Num), Adaptive Law A_T #2/1(Agent_Num), Adaptive Law g_T #2/1(Agent_Num)
  Ti/1 -> Adaptive Law A_T #2/3(T_i), Module to compute Consensus Error_T #2/1(T_i), Main Controller_T #2/8(T_i)
  x0_hati/1 -> Adaptive Law A_T #2/7(x0_hat_inp), Main Controller_T #2/12(x0_hat_inp)
  DTi/1 -> Main Controller_T #2/7(DT_i)
  qi/1 -> Main Controller_T #2/9(q_i)
  Differentiator1/1(Dx_d) -> Main Controller_T #2/14(D_ui1)

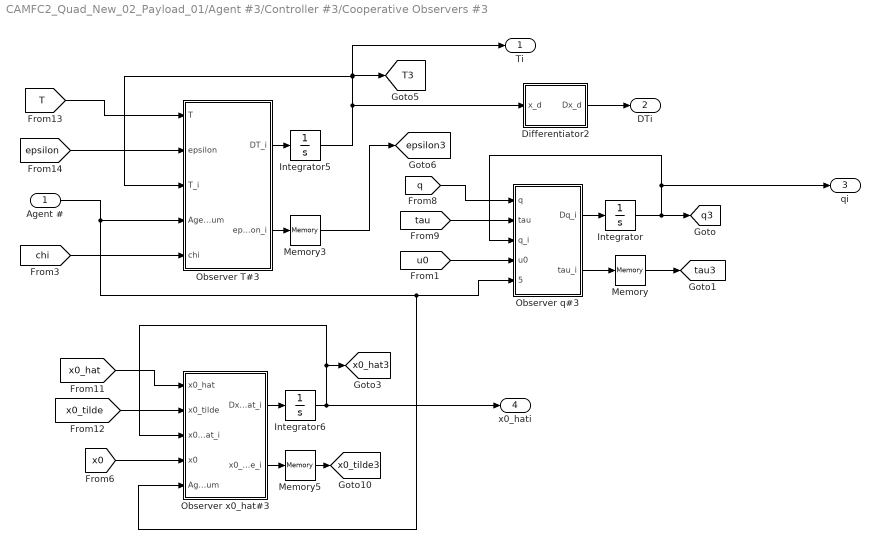
== system CAMFC2_Quad_New_02_Payload_01/Agent #3/Controller #3/Cooperative Observers #3 ==
  Agent # : Inport
  Differentiator2 : Subsystem
  Integrator : Integrator  InitialCondition=zeros(n0,1)
  Integrator5 : Integrator  InitialCondition=zeros(N+1,n0)
  Integrator6 : Integrator  InitialCondition=zeros(n0,1)
  Memory : Memory  InitialCondition=zeros(n0,1)
  Memory3 : Memory  InitialCondition=zeros(N+1,n0)
  Memory5 : Memory  InitialCondition=zeros(n0,1)
  Observer T#3 : MATLAB Function  TreatAsAtomicUnit=on
  Observer q#3 : MATLAB Function  TreatAsAtomicUnit=on
  Observer x0_hat#3 : MATLAB Function  TreatAsAtomicUnit=on
  Ti : Outport
  DTi : Outport  Port=2
  qi : Outport  Port=3
  x0_hati : Outport  Port=4
  tag scope: T3=global, epsilon3=global, q3=global, tau3=global, x0_hat3=global, x0_tilde3=global
  wires:
  [x0_tilde] -> Observer x0_hat#3/2(x0_tilde)
  Agent #/1 -> Observer q#3/5(Agent_Num), Observer x0_hat#3/5(Agent_Num), Observer T#3/4(Agent_Num)
  Observer T#3/1(DT_i) -> Integrator5/1
  Integrator/1 -> [q3], qi/1, Observer q#3/3(q_i)
  [q] -> Observer q#3/1(q)
  Observer q#3/1(Dq_i) -> Integrator/1
  Observer T#3/2(epsilon_i) -> Memory3/1
  [x0] -> Observer x0_hat#3/4(x0)
  [x0_hat] -> Observer x0_hat#3/1(x0_hat)
  [chi] -> Observer T#3/5(chi)
  Integrator5/1 -> Ti/1, [T3], Observer T#3/3(T_i), Differentiator2/1(x_d)
  [T] -> Observer T#3/1(T)
  Observer x0_hat#3/1(Dx0_hat_i) -> Integrator6/1
  [epsilon] -> Observer T#3/2(epsilon)
  [tau] -> Observer q#3/2(tau)
  Memory5/1 -> [x0_tilde3]
  Observer x0_hat#3/2(x0_tilde_i) -> Memory5/1
  Integrator6/1 -> x0_hati/1, Observer x0_hat#3/3(x0_hat_i), [x0_hat3]
  Memory3/1 -> [epsilon3]
  Memory/1 -> [tau3]
  Observer q#3/2(tau_i) -> Memory/1
  [u0] -> Observer q#3/4(u0)
  Differentiator2/1(Dx_d) -> DTi/1

== system CAMFC2_Quad_New_02_Payload_01/Agent #3/Controller #3/Rotational ==
  x_rd : Inport
  X : Inport  Port=2
  CARE : MATLAB Function  TreatAsAtomicUnit=on
  Differentiator : Subsystem
  Integrator : Integrator  InitialCondition=zeros(n)
  Integrator1 : Integrator  InitialCondition=eye(n)
  Integrator2 : Integrator  InitialCondition=zeros(n,1)
  Integrator3 : Integrator  InitialCondition=zeros(n,1)
  Memory : Memory  InitialCondition=zeros(m,1)
  Scope10 : Scope
  Sum : Sum  Inputs=|++
  g-Estimator : MATLAB Function  TreatAsAtomicUnit=on
  g-Estimator1 : MATLAB Function  TreatAsAtomicUnit=on
  main : MATLAB Function  TreatAsAtomicUnit=on
  variable change : MATLAB Function  TreatAsAtomicUnit=on
  ur : Outport
  tag scope: A_hat3_R=global, P3_R=global, e3_R=global, g_hat3_R=global
  wires:
  x_rd/1 -> variable change/2(Xd)
  X/1 -> variable change/1(X)
  CARE/1(DP) -> Integrator1/1
  Sum/1 -> main/1(sigma), Scope10/1, g-Estimator/1(sigma), g-Estimator1/1(sigma)
  g-Estimator1/1(Da_hat) -> Integrator/1
  variable change/1(x_mod) -> main/7(x), g-Estimator1/2(x)
  Integrator1/1 -> g-Estimator1/3(P), CARE/1(P), [P3_R], g-Estimator/3(P), main/4(P)
  Integrator/1 -> [A_hat3_R], g-Estimator1/4(a_hat), CARE/2(a_hat), main/5(a_hat)
  g-Estimator/1(Dg_hat) -> Integrator2/1
  Differentiator/1(Dx_d) -> main/3(Dy_d)
  main/1(u) -> Memory/1, ur/1
  Integrator3/1 -> main/2(zeta), Sum/1
  variable change/2(xd_mod) -> Differentiator/1(x_d)
  variable change/3(e_mod) -> [e3_R], Sum/2, Integrator3/1
  Memory/1 -> variable change/3(u)
  Integrator2/1 -> [g_hat3_R], main/6(g_hat), g-Estimator/2(g_hat)

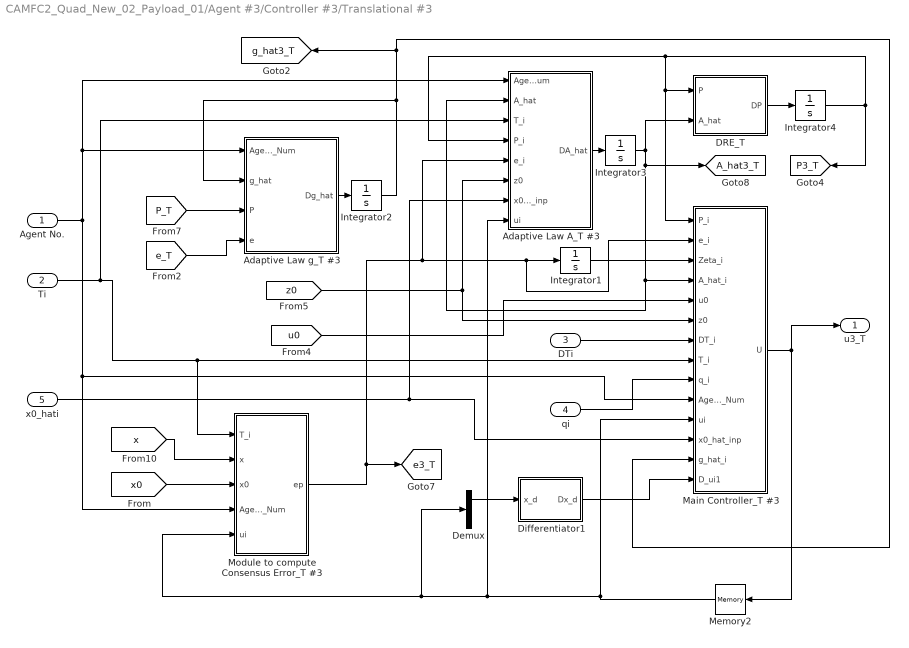
== system CAMFC2_Quad_New_02_Payload_01/Agent #3/Controller #3/Translational #3 ==
  Agent No. : Inport
  Ti : Inport  Port=2
  DTi : Inport  Port=3
  qi : Inport  Port=4
  x0_hati : Inport  Port=5
  Adaptive Law A_T #3 : MATLAB Function  TreatAsAtomicUnit=on
  Adaptive Law g_T #3 : MATLAB Function  TreatAsAtomicUnit=on
  DRE_T : MATLAB Function  TreatAsAtomicUnit=on
  Demux : Demux  Outputs=2
  Differentiator1 : Subsystem
  Integrator1 : Integrator  InitialCondition=zeros(n,1)
  Integrator2 : Integrator  InitialCondition=zeros(n,1)
  Integrator3 : Integrator  InitialCondition=zeros(n)
  Integrator4 : Integrator  InitialCondition=eye(n)
  Main Controller_T #3 : MATLAB Function  TreatAsAtomicUnit=on
  Memory2 : Memory  InitialCondition=zeros(n,1)
  Module to compute Consensus Error_T #3 : MATLAB Function  TreatAsAtomicUnit=on
  u3_T : Outport
  tag scope: A_hat3_T=global, P3_T=global, e3_T=global, g_hat3_T=global
  wires:
  [u0] -> Main Controller_T #3/5(u0)
  DRE_T/1(DP) -> Integrator4/1
  Module to compute Consensus Error_T #3/1(ep) -> Adaptive Law A_T #3/5(e_i), Main Controller_T #3/2(e_i), Integrator1/1, [e3_T]
  Adaptive Law g_T #3/1(Dg_hat) -> Integrator2/1
  Demux/1 -> Differentiator1/1(x_d)
  Main Controller_T #3/1(U) -> u3_T/1, Memory2/1
  Memory2/1 -> Main Controller_T #3/11(ui), Adaptive Law A_T #3/8(ui), Module to compute Consensus Error_T #3/5(ui), Demux/1
  Adaptive Law A_T #3/1(DA_hat) -> Integrator3/1
  Integrator2/1 -> Main Controller_T #3/13(g_hat_i), [g_hat3_T], Adaptive Law g_T #3/2(g_hat)
  [e_T] -> Adaptive Law g_T #3/4(e)
  Integrator1/1 -> Main Controller_T #3/3(Zeta_i)
  Integrator3/1 -> [A_hat3_T], Adaptive Law A_T #3/2(A_hat), Main Controller_T #3/4(A_hat_i), DRE_T/2(A_hat)
  Integrator4/1 -> [P3_T], Adaptive Law A_T #3/4(P_i), DRE_T/1(P), Main Controller_T #3/1(P_i)
  [P_T] -> Adaptive Law g_T #3/3(P)
  [x0] -> Module to compute Consensus Error_T #3/3(x0)
  [x] -> Module to compute Consensus Error_T #3/2(x)
  [z0] -> Adaptive Law A_T #3/6(z0), Main Controller_T #3/6(z0)
  Agent No./1 -> Main Controller_T #3/10(Agent_Num), Module to compute Consensus Error_T #3/4(Agent_Num), Adaptive Law A_T #3/1(Agent_Num), Adaptive Law g_T #3/1(Agent_Num)
  Ti/1 -> Adaptive Law A_T #3/3(T_i), Module to compute Consensus Error_T #3/1(T_i), Main Controller_T #3/8(T_i)
  x0_hati/1 -> Adaptive Law A_T #3/7(x0_hat_inp), Main Controller_T #3/12(x0_hat_inp)
  DTi/1 -> Main Controller_T #3/7(DT_i)
  qi/1 -> Main Controller_T #3/9(q_i)
  Differentiator1/1(Dx_d) -> Main Controller_T #3/14(D_ui1)

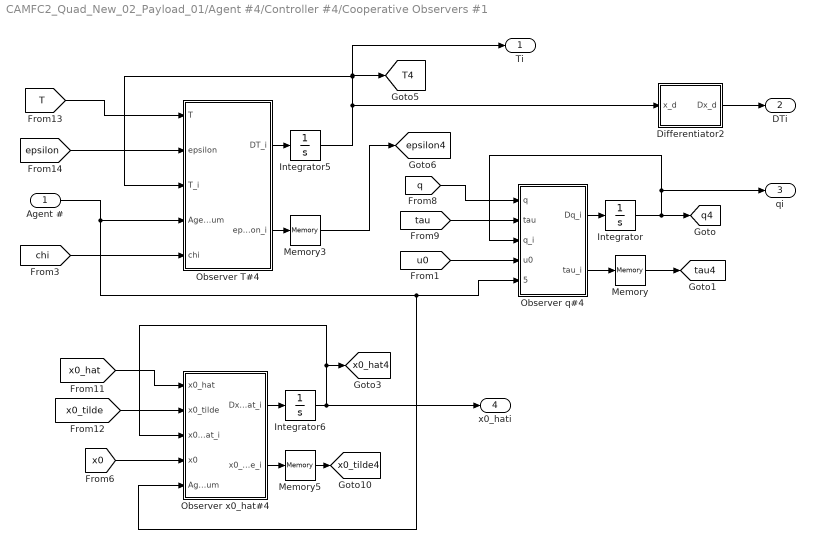
== system CAMFC2_Quad_New_02_Payload_01/Agent #4/Controller #4/Cooperative Observers #1 ==
  Agent # : Inport
  Differentiator2 : Subsystem
  Integrator : Integrator  InitialCondition=zeros(n0,1)
  Integrator5 : Integrator  InitialCondition=zeros(N+1,n0)
  Integrator6 : Integrator  InitialCondition=zeros(n0,1)
  Memory : Memory  InitialCondition=zeros(n0,1)
  Memory3 : Memory  InitialCondition=zeros(N+1,n0)
  Memory5 : Memory  InitialCondition=zeros(n0,1)
  Observer T#4 : MATLAB Function  TreatAsAtomicUnit=on
  Observer q#4 : MATLAB Function  TreatAsAtomicUnit=on
  Observer x0_hat#4 : MATLAB Function  TreatAsAtomicUnit=on
  Ti : Outport
  DTi : Outport  Port=2
  qi : Outport  Port=3
  x0_hati : Outport  Port=4
  tag scope: T4=global, epsilon4=global, q4=global, tau4=global, x0_hat4=global, x0_tilde4=global
  wires:
  [x0_tilde] -> Observer x0_hat#4/2(x0_tilde)
  Agent #/1 -> Observer q#4/5(Agent_Num), Observer x0_hat#4/5(Agent_Num), Observer T#4/4(Agent_Num)
  Observer T#4/1(DT_i) -> Integrator5/1
  Integrator/1 -> [q4], qi/1, Observer q#4/3(q_i)
  [q] -> Observer q#4/1(q)
  Observer q#4/1(Dq_i) -> Integrator/1
  Observer T#4/2(epsilon_i) -> Memory3/1
  [x0] -> Observer x0_hat#4/4(x0)
  [x0_hat] -> Observer x0_hat#4/1(x0_hat)
  [chi] -> Observer T#4/5(chi)
  Integrator5/1 -> Ti/1, [T4], Observer T#4/3(T_i), Differentiator2/1(x_d)
  [T] -> Observer T#4/1(T)
  Observer x0_hat#4/1(Dx0_hat_i) -> Integrator6/1
  [epsilon] -> Observer T#4/2(epsilon)
  [tau] -> Observer q#4/2(tau)
  Memory5/1 -> [x0_tilde4]
  Observer x0_hat#4/2(x0_tilde_i) -> Memory5/1
  Integrator6/1 -> x0_hati/1, Observer x0_hat#4/3(x0_hat_i), [x0_hat4]
  Memory3/1 -> [epsilon4]
  Memory/1 -> [tau4]
  Observer q#4/2(tau_i) -> Memory/1
  [u0] -> Observer q#4/4(u0)
  Differentiator2/1(Dx_d) -> DTi/1

== system CAMFC2_Quad_New_02_Payload_01/Agent #4/Controller #4/Rotational ==
  x_rd : Inport
  X : Inport  Port=2
  CARE : MATLAB Function  TreatAsAtomicUnit=on
  Differentiator : Subsystem
  Integrator : Integrator  InitialCondition=zeros(n)
  Integrator1 : Integrator  InitialCondition=eye(n)
  Integrator2 : Integrator  InitialCondition=zeros(n,1)
  Integrator3 : Integrator  InitialCondition=zeros(n,1)
  Memory : Memory  InitialCondition=zeros(m,1)
  Scope10 : Scope
  Sum : Sum  Inputs=|++
  g-Estimator : MATLAB Function  TreatAsAtomicUnit=on
  g-Estimator1 : MATLAB Function  TreatAsAtomicUnit=on
  main : MATLAB Function  TreatAsAtomicUnit=on
  variable change : MATLAB Function  TreatAsAtomicUnit=on
  ur : Outport
  tag scope: A_hat4_R=global, P4_R=global, e4_R=global, g_hat4_R=global
  wires:
  x_rd/1 -> variable change/2(Xd)
  X/1 -> variable change/1(X)
  CARE/1(DP) -> Integrator1/1
  Sum/1 -> main/1(sigma), Scope10/1, g-Estimator/1(sigma), g-Estimator1/1(sigma)
  g-Estimator1/1(Da_hat) -> Integrator/1
  variable change/1(x_mod) -> main/7(x), g-Estimator1/2(x)
  Integrator1/1 -> g-Estimator1/3(P), CARE/1(P), [P4_R], g-Estimator/3(P), main/4(P)
  Integrator/1 -> [A_hat4_R], g-Estimator1/4(a_hat), CARE/2(a_hat), main/5(a_hat)
  g-Estimator/1(Dg_hat) -> Integrator2/1
  Differentiator/1(Dx_d) -> main/3(Dy_d)
  main/1(u) -> Memory/1, ur/1
  Integrator3/1 -> main/2(zeta), Sum/1
  variable change/2(xd_mod) -> Differentiator/1(x_d)
  variable change/3(e_mod) -> [e4_R], Sum/2, Integrator3/1
  Memory/1 -> variable change/3(u)
  Integrator2/1 -> [g_hat4_R], main/6(g_hat), g-Estimator/2(g_hat)

== system CAMFC2_Quad_New_02_Payload_01/Agent #4/Controller #4/Translational #4 ==
  Agent No. : Inport
  Ti : Inport  Port=2
  DTi : Inport  Port=3
  qi : Inport  Port=4
  x0_hati : Inport  Port=5
  Adaptive Law A_T #4 : MATLAB Function  TreatAsAtomicUnit=on
  Adaptive Law g_T #4 : MATLAB Function  TreatAsAtomicUnit=on
  DRE_T : MATLAB Function  TreatAsAtomicUnit=on
  Demux : Demux  Outputs=2
  Differentiator1 : Subsystem
  Integrator1 : Integrator  InitialCondition=zeros(n,1)
  Integrator2 : Integrator  InitialCondition=zeros(n,1)
  Integrator3 : Integrator  InitialCondition=zeros(n)
  Integrator4 : Integrator  InitialCondition=eye(n)
  Main Controller_T #4 : MATLAB Function  TreatAsAtomicUnit=on
  Memory2 : Memory  InitialCondition=zeros(n,1)
  Module to compute Consensus Error_T #4 : MATLAB Function  TreatAsAtomicUnit=on
  u4_T : Outport
  tag scope: A_hat4_T=global, P4_T=global, e4_T=global, g_hat4_T=global
  wires:
  [u0] -> Main Controller_T #4/5(u0)
  DRE_T/1(DP) -> Integrator4/1
  Module to compute Consensus Error_T #4/1(ep) -> Adaptive Law A_T #4/5(e_i), Main Controller_T #4/2(e_i), Integrator1/1, [e4_T]
  Adaptive Law g_T #4/1(Dg_hat) -> Integrator2/1
  Demux/1 -> Differentiator1/1(x_d)
  Main Controller_T #4/1(U) -> u4_T/1, Memory2/1
  Memory2/1 -> Module to compute Consensus Error_T #4/5(ui), Demux/1, Adaptive Law A_T #4/8(ui), Main Controller_T #4/11(ui)
  Adaptive Law A_T #4/1(DA_hat) -> Integrator3/1
  Integrator2/1 -> Main Controller_T #4/13(g_hat_i), [g_hat4_T], Adaptive Law g_T #4/2(g_hat)
  [e_T] -> Adaptive Law g_T #4/4(e)
  Integrator1/1 -> Main Controller_T #4/3(Zeta_i)
  Integrator3/1 -> [A_hat4_T], Adaptive Law A_T #4/2(A_hat), Main Controller_T #4/4(A_hat_i), DRE_T/2(A_hat)
  Integrator4/1 -> [P4_T], Adaptive Law A_T #4/4(P_i), DRE_T/1(P), Main Controller_T #4/1(P_i)
  [P_T] -> Adaptive Law g_T #4/3(P)
  [x0] -> Module to compute Consensus Error_T #4/3(x0)
  [x] -> Module to compute Consensus Error_T #4/2(x)
  [z0] -> Adaptive Law A_T #4/6(z0), Main Controller_T #4/6(z0)
  Agent No./1 -> Main Controller_T #4/10(Agent_Num), Module to compute Consensus Error_T #4/4(Agent_Num), Adaptive Law A_T #4/1(Agent_Num), Adaptive Law g_T #4/1(Agent_Num)
  Ti/1 -> Adaptive Law A_T #4/3(T_i), Module to compute Consensus Error_T #4/1(T_i), Main Controller_T #4/8(T_i)
  x0_hati/1 -> Adaptive Law A_T #4/7(x0_hat_inp), Main Controller_T #4/12(x0_hat_inp)
  DTi/1 -> Main Controller_T #4/7(DT_i)
  qi/1 -> Main Controller_T #4/9(q_i)
  Differentiator1/1(Dx_d) -> Main Controller_T #4/14(D_ui1)

== system CAMFC2_Quad_New_02_Payload_01/Data Bus /Observers Log/For matrix Plot10 ==
  T : Inport
  MATLAB Function : MATLAB Function  TreatAsAtomicUnit=on
  To Workspace : ToWorkspace  VariableName=T3  SaveFormat=Structure With Time  SampleTime=-1
  wires:
  T/1 -> MATLAB Function/1(u)
  MATLAB Function/1(y) -> To Workspace/1

== system CAMFC2_Quad_New_02_Payload_01/Data Bus /Observers Log/For matrix Plot11 ==
  T : Inport
  MATLAB Function : MATLAB Function  TreatAsAtomicUnit=on
  To Workspace : ToWorkspace  VariableName=T4  SaveFormat=Structure With Time  SampleTime=-1
  wires:
  MATLAB Function/1(y) -> To Workspace/1
  T/1 -> MATLAB Function/1(u)

== system CAMFC2_Quad_New_02_Payload_01/Data Bus /Observers Log/For matrix Plot12 ==
  epsilon : Inport
  MATLAB Function : MATLAB Function  TreatAsAtomicUnit=on
  To Workspace : ToWorkspace  VariableName=epsilon1  SaveFormat=Structure With Time  SampleTime=-1
  wires:
  epsilon/1 -> MATLAB Function/1(u)
  MATLAB Function/1(y) -> To Workspace/1

== system CAMFC2_Quad_New_02_Payload_01/Data Bus /Observers Log/For matrix Plot13 ==
  epsilon : Inport
  MATLAB Function : MATLAB Function  TreatAsAtomicUnit=on
  To Workspace : ToWorkspace  VariableName=epsilon2  SaveFormat=Structure With Time  SampleTime=-1
  wires:
  MATLAB Function/1(y) -> To Workspace/1
  epsilon/1 -> MATLAB Function/1(u)

== system CAMFC2_Quad_New_02_Payload_01/Data Bus /Observers Log/For matrix Plot14 ==
  epsilon : Inport
  MATLAB Function : MATLAB Function  TreatAsAtomicUnit=on
  To Workspace : ToWorkspace  VariableName=epsilon3  SaveFormat=Structure With Time  SampleTime=-1
  wires:
  MATLAB Function/1(y) -> To Workspace/1
  epsilon/1 -> MATLAB Function/1(u)

== system CAMFC2_Quad_New_02_Payload_01/Data Bus /Observers Log/For matrix Plot15 ==
  epsilon : Inport
  MATLAB Function : MATLAB Function  TreatAsAtomicUnit=on
  To Workspace : ToWorkspace  VariableName=epsilon4  SaveFormat=Structure With Time  SampleTime=-1
  wires:
  epsilon/1 -> MATLAB Function/1(u)
  MATLAB Function/1(y) -> To Workspace/1

== system CAMFC2_Quad_New_02_Payload_01/Data Bus /Observers Log/For matrix Plot8 ==
  T : Inport
  MATLAB Function : MATLAB Function  TreatAsAtomicUnit=on
  To Workspace : ToWorkspace  VariableName=T1  SaveFormat=Structure With Time  SampleTime=-1
  wires:
  MATLAB Function/1(y) -> To Workspace/1
  T/1 -> MATLAB Function/1(u)

== system CAMFC2_Quad_New_02_Payload_01/Data Bus /Observers Log/For matrix Plot9 ==
  T : Inport
  MATLAB Function : MATLAB Function  TreatAsAtomicUnit=on
  To Workspace : ToWorkspace  VariableName=T2  SaveFormat=Structure With Time  SampleTime=-1
  wires:
  T/1 -> MATLAB Function/1(u)
  MATLAB Function/1(y) -> To Workspace/1
